simulink model "test2"  (R2020a)
settings: Solver=VariableStepAuto  StartTime=0.0  StopTime=10.0  RelTol=1e-3
libraries: simulink x1
settings Model: Creator=HP  LastModifiedBy=86150
settings DataIOCC: ReturnWorkspaceOutputs=off
settings DebuggingCC: ArithmeticOperatorsInVariantConditions=warning
settings SFSimCC: CustomCodeUndefinedFunction=UseInterfaceOnly

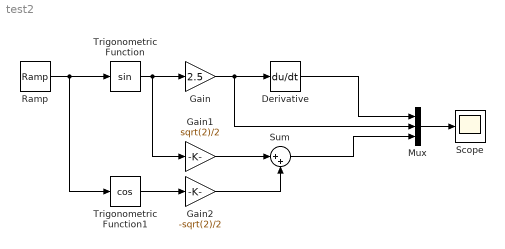
== system test2 ==
  Derivative : Derivative
  Gain : Gain  Gain=2.5
  Gain1 : Gain  Gain=sqrt(2)/2
  Gain2 : Gain  Gain=-sqrt(2)/2
  Mux : Mux  Inputs=3
  Ramp : simulink/Sources/Ramp  slope=1  start=0  InitialOutput=0  VectorParams1D=off
  Scope : Scope
  Sum : Sum  Inputs=|++
  Trigonometric Function : Trigonometry
  Trigonometric Function1 : Trigonometry  Operator=cos
  wires:
  Ramp/1 -> Trigonometric Function1/1, Trigonometric Function/1
  Gain/1 -> Derivative/1, Mux/2
  Trigonometric Function/1 -> Gain1/1, Gain/1
  Trigonometric Function1/1 -> Gain2/1
  Gain1/1 -> Sum/1
  Gain2/1 -> Sum/2
  Sum/1 -> Mux/3
  Mux/1 -> Scope/1
  Derivative/1 -> Mux/1
